simulink model "closed_loop5"  (R2012b)
settings: Solver=ode3  StartTime=0.0  StopTime=t_total+100  FixedStep=0.001  RelTol=1e-3
values from neighbouring files (symbols this model uses):
  a = D/(8*(t1^2)*(n^2))    [Craneparameters.m]    (also in Craneparameters2.m = 0.428041999052; Craneparameters3.m = 0.428041999052; Craneparameters4.m = 0.5; Craneparameters5.m = 0.428041999052)
  a2 = D/(2*(4*p+1)*p*(t1^2))    [Craneparameters2.m]    (also in Craneparameters3.m = D/(2*(4*n+5)*(n+1)*(t1^2)); Craneparameters5.m = D/(2*(4*n+5)*(n+1)*(t1^2)))
  g = 9.81    [Craneparameters.m]    (also in Craneparameters2.m; Craneparameters3.m; Craneparameters4.m; Craneparameters5.m)
  K = 2/w    [Craneparameters4.m]    (also in Craneparameters5.m; Prototype_parameters.m; Slidingmode.m)
  l = 40    [Craneparameters.m]    (also in Craneparameters2.m; Craneparameters3.m; Craneparameters4.m; Craneparameters5.m)
  M = 26*10^3    (= 26000)    [Craneparameters.m]    (also in Craneparameters2.m; Craneparameters3.m; Craneparameters4.m; Craneparameters5.m)
  m = 67.3*10^3    (= 67300)    [Craneparameters.m]    (also in Craneparameters2.m; Craneparameters3.m; Craneparameters4.m; Craneparameters5.m)
  T = 2*pi/w    [Craneparameters.m]    (also in Craneparameters2.m; Craneparameters3.m; Craneparameters4.m; Craneparameters5.m)
  T1 = n*T    [Craneparameters.m]    (also in Craneparameters2.m; Craneparameters3.m; Craneparameters4.m = t1; Craneparameters5.m)
  T2 = n*T+t2    [Craneparameters.m]    (also in Craneparameters2.m; Craneparameters3.m = (n+1)*T; Craneparameters4.m = t1+t2; Craneparameters5.m = (n+1)*T)
  T3 = (n+1)*T+t2    [Craneparameters3.m]    (also in Craneparameters5.m)
  T4 = (n+2)*T+t2    [Craneparameters3.m]    (also in Craneparameters5.m)
  t_total = 2*n*T + t2    [Craneparameters.m]    (also in Craneparameters2.m = t_total2; Craneparameters3.m = 2*(n+1)*T + t2; Craneparameters4.m = T2+t1; Craneparameters5.m = 2*(n+1)*T + t2)
libraries: simulink x2
settings Model: Creator=mchusr  LastModifiedBy=mchusr

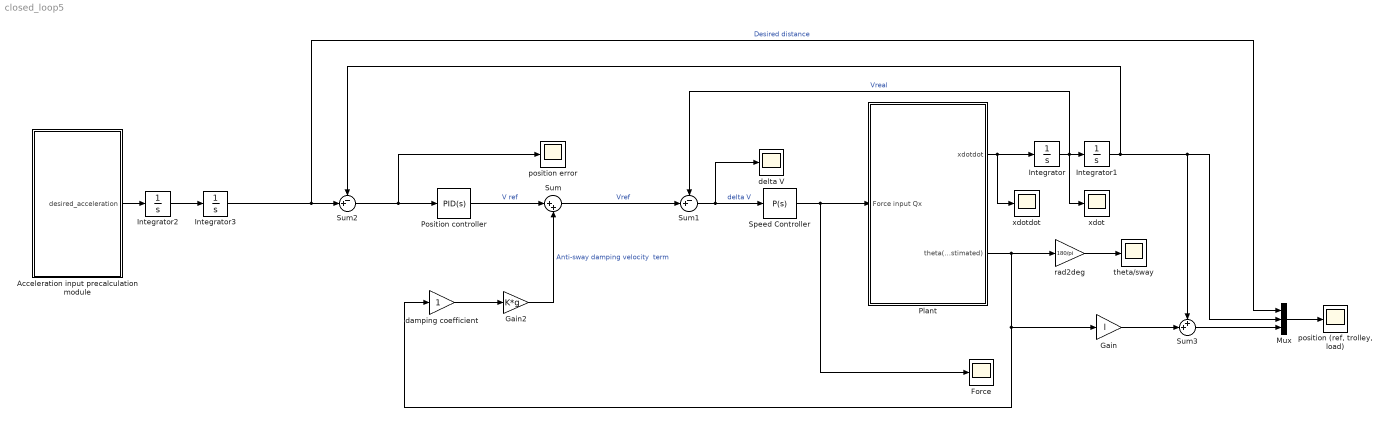
== system closed_loop5 ==
  Acceleration input precalculation module : Subsystem
  Force : Scope
      settings: TimeRange=105  YMin=-600000  YMax=100000  SaveName=xdotdot1
  Gain : Gain  Gain=l
  Gain2 : Gain  Gain=K*g
  Integrator{,1..3} (4 alike) : Integrator
  Mux : Mux  Inputs=3
  Plant : Subsystem
  Position controller : simulink/Continuous/PID Controller  Controller=PID  TimeDomain=Continuous-time  SampleTime=1  IntegratorMethod=Forward Euler  FilterMethod=Forward Euler  Form=Parallel  P=3  I=0.08  D=0.4  N=100  InitialConditionSource=internal  InitialConditionForIntegrator=0  InitialConditionForFilter=0  ExternalReset=none  LimitOutput=off  UpperSaturationLimit=inf  LowerSaturationLimit=-inf  LinearizeAsGain=on  AntiWindupMode=none  Kb=1  TrackingMode=off  Kt=1  PParamMin=[]  PParamMax=[]  IParamMin=[]  IParamMax=[]  DParamMin=[]  DParamMax=[]  NParamMin=[]  NParamMax=[]  KbParamMin=[]  KbParamMax=[]  KtParamMin=[]  KtParamMax=[]  POutMin=[]  POutMax=[]  IOutMin=[]  IOutMax=[]  DOutMin=[]  DOutMax=[]  NOutMin=[]  NOutMax=[]  KbOutMin=[]  KbOutMax=[]  KtOutMin=[]  KtOutMax=[]  IntegratorOutMin=[]  IntegratorOutMax=[]  FilterOutMin=[]  FilterOutMax=[]  SumOutMin=[]  SumOutMax=[]  SumI1OutMin=[]  SumI1OutMax=[]  SumI2OutMin=[]  SumI2OutMax=[]  SumI3OutMin=[]  SumI3OutMax=[]  SumDOutMin=[]  SumDOutMax=[]  SaturationOutMin=[]  SaturationOutMax=[]  IntegratorContinuousStateAttributes=''  IntegratorStateMustResolveToSignalObject=off  IntegratorRTWStateStorageClass=Auto  FilterContinuousStateAttributes=''  FilterStateMustResolveToSignalObject=off  FilterRTWStateStorageClass=Auto
  Speed Controller : simulink/Continuous/PID Controller  Controller=P  TimeDomain=Continuous-time  SampleTime=1  IntegratorMethod=Forward Euler  FilterMethod=Forward Euler  Form=Parallel  P=(M+m)  I=10*(M+m)  D=(M+m)  N=100  InitialConditionSource=internal  InitialConditionForIntegrator=0  InitialConditionForFilter=0  ExternalReset=none  LimitOutput=off  UpperSaturationLimit=inf  LowerSaturationLimit=-inf  LinearizeAsGain=on  AntiWindupMode=none  Kb=1  TrackingMode=off  Kt=1  PParamMin=[]  PParamMax=[]  IParamMin=[]  IParamMax=[]  DParamMin=[]  DParamMax=[]  NParamMin=[]  NParamMax=[]  KbParamMin=[]  KbParamMax=[]  KtParamMin=[]  KtParamMax=[]  POutMin=[]  POutMax=[]  IOutMin=[]  IOutMax=[]  DOutMin=[]  DOutMax=[]  NOutMin=[]  NOutMax=[]  KbOutMin=[]  KbOutMax=[]  KtOutMin=[]  KtOutMax=[]  IntegratorOutMin=[]  IntegratorOutMax=[]  FilterOutMin=[]  FilterOutMax=[]  SumOutMin=[]  SumOutMax=[]  SumI1OutMin=[]  SumI1OutMax=[]  SumI2OutMin=[]  SumI2OutMax=[]  SumI3OutMin=[]  SumI3OutMax=[]  SumDOutMin=[]  SumDOutMax=[]  SaturationOutMin=[]  SaturationOutMax=[]  IntegratorContinuousStateAttributes=''  IntegratorStateMustResolveToSignalObject=off  IntegratorRTWStateStorageClass=Auto  FilterContinuousStateAttributes=''  FilterStateMustResolveToSignalObject=off  FilterRTWStateStorageClass=Auto
  Sum : Sum  Inputs=|++
  Sum1 : Sum  Inputs=-+|
  Sum2 : Sum  Inputs=-+|
  Sum3 : Sum  Inputs=++|
  damping coefficient : Gain
  delta V : Scope
      settings: TimeRange=105  YMin=-7.5e-08  YMax=7.5e-08  SaveName=xdotdot3
  "position (ref, trolley, load)" : Scope
      settings: TimeRange=139.097  YMin=98.25  YMax=101.75  SaveName=position2
  position error : Scope
      settings: TimeRange=105  YMin=-0.105  YMax=-0.025  SaveName=xdotdot2
  rad2deg : Gain  Gain=180/pi
  theta/sway : Scope
      settings: YMin=-0.175  YMax=0.175  SaveName=sway2
  xdot : Scope
      settings: TimeRange=64.833  YMin=5.55112e-17  YMax=1.9  SaveName=velocity
  xdotdot : Scope
      settings: TimeRange=105  YMin=-7.5e-08  YMax=7.5e-08  SaveName=xdotdot
  wires:
  Plant/1(xdotdot) -> Integrator/1, xdotdot/1
  Integrator/1 -> Sum1/1, xdot/1, Integrator1/1  "Vreal"
  Integrator1/1 -> Mux/2, Sum3/1, Sum2/1
  Plant/2(theta(estimated)) -> rad2deg/1, damping coefficient/1, Gain/1
  Speed Controller/1 -> Plant/1(Force input Qx), Force/1
  Position controller/1 -> Sum/1  "V ref"
  Gain2/1 -> Sum/2  "Anti-sway damping velocity  term"
  damping coefficient/1 -> Gain2/1
  Sum/1 -> Sum1/2  "Vref"
  Sum1/1 -> delta V/1, Speed Controller/1  "delta V"
  Sum2/1 -> position error/1, Position controller/1
  Integrator3/1 -> Sum2/2, Mux/1  "Desired distance"
  rad2deg/1 -> theta/sway/1
  Gain/1 -> Sum3/2
  Sum3/1 -> Mux/3
  Mux/1 -> "position (ref, trolley, load)"/1
  Acceleration input precalculation module/1(desired_acceleration) -> Integrator2/1
  Integrator2/1 -> Integrator3/1

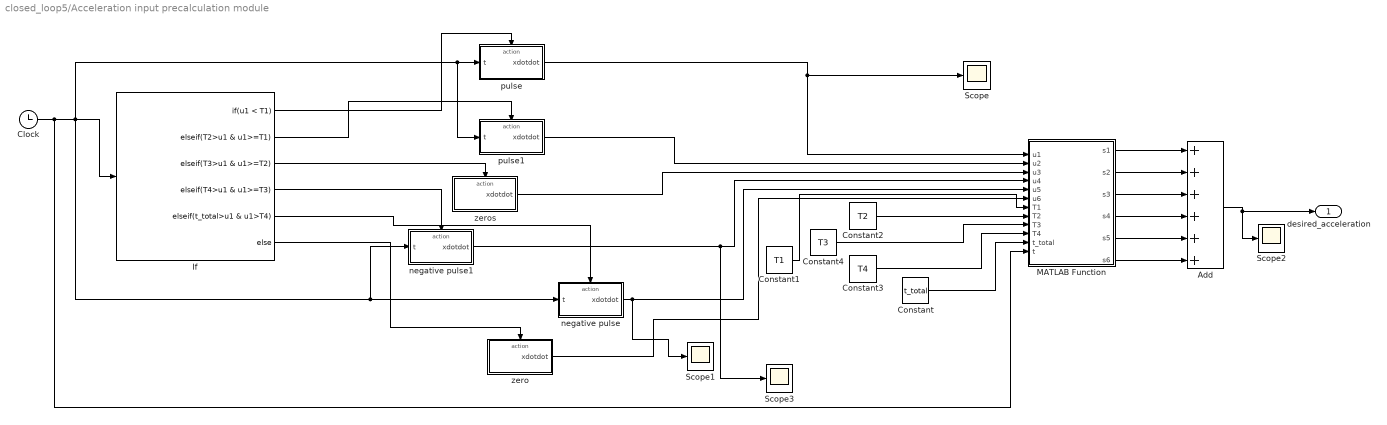
== system closed_loop5/Acceleration input precalculation module ==
  Add : Sum  Inputs=++++++
  Clock : Clock
  Constant : Constant  Value=t_total
  Constant1 : Constant  Value=T1
  Constant2 : Constant  Value=T2
  Constant3 : Constant  Value=T4
  Constant4 : Constant  Value=T3
  If : If  IfExpression=u1 < T1  ElseIfExpressions=T2>u1 & u1>=T1, T3>u1 & u1>=T2, T4>u1 & u1>=T3, t_total>u1 & u1>T4  ZeroCross=off
  MATLAB Function : MATLAB Function  TreatAsAtomicUnit=on
  Scope{,1..3} (4 alike) : Scope
      Scope settings: SaveName=ScopeData4
      Scope1 settings: SaveName=ScopeData5
      Scope2 settings: SaveName=ScopeData6
  negative pulse : Subsystem  TreatAsAtomicUnit=on
  negative pulse1 : Subsystem  TreatAsAtomicUnit=on
  pulse : Subsystem  TreatAsAtomicUnit=on
  pulse1 : Subsystem  TreatAsAtomicUnit=on
  "zero " : Subsystem  TreatAsAtomicUnit=on
  zeros : Subsystem  TreatAsAtomicUnit=on
  desired_acceleration : Outport
  wires:
  If/1 -> pulse/Action
  Clock/1 -> MATLAB Function/12(t), pulse1/1(t), pulse/1(t), negative pulse1/1(t), negative pulse/1(t), If/1
  Add/1 -> Scope2/1, desired_acceleration/1
  pulse/1(xdotdot) -> MATLAB Function/1(u1), Scope/1
  MATLAB Function/1(s1) -> Add/1
  MATLAB Function/2(s2) -> Add/2
  MATLAB Function/3(s3) -> Add/3
  MATLAB Function/4(s4) -> Add/4
  Constant1/1 -> MATLAB Function/7(T1)
  Constant/1 -> MATLAB Function/11(t_total)
  MATLAB Function/5(s5) -> Add/5
  Constant2/1 -> MATLAB Function/8(T2)
  Constant4/1 -> MATLAB Function/9(T3)
  Constant3/1 -> MATLAB Function/10(T4)
  If/2 -> pulse1/Action
  pulse1/1(xdotdot) -> MATLAB Function/2(u2)
  If/3 -> zeros/Action
  zeros/1(xdotdot) -> MATLAB Function/3(u3)
  If/4 -> negative pulse1/Action
  If/5 -> negative pulse/Action
  negative pulse1/1(xdotdot) -> Scope3/1, MATLAB Function/4(u4)
  negative pulse/1(xdotdot) -> Scope1/1, MATLAB Function/5(u5)
  If/6 -> "zero "/Action
  "zero "/1(xdotdot) -> MATLAB Function/6(u6)
  MATLAB Function/6(s6) -> Add/6

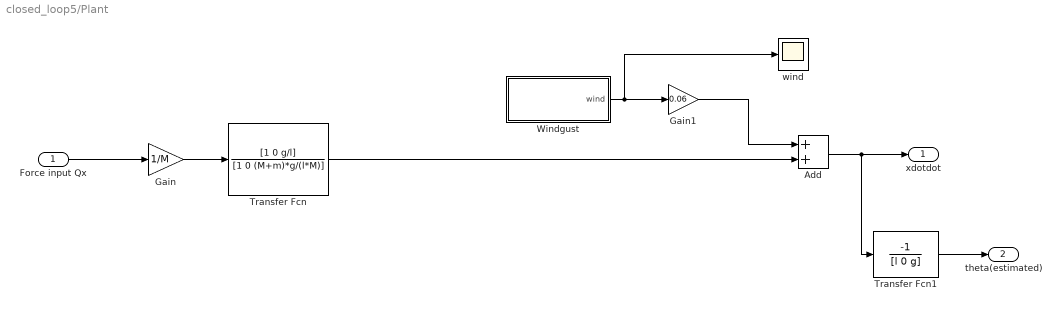
== system closed_loop5/Plant ==
  Force input Qx : Inport
  Add : Sum
  Gain : Gain  Gain=1/M
  Gain1 : Gain  Gain=0.06
  Transfer Fcn : TransferFcn  Numerator=[1 0 g/l]  Denominator=[1 0 (M+m)*g/(l*M)]
  Transfer Fcn1 : TransferFcn  Numerator=[-1]  Denominator=[l 0 g]
  Windgust : Subsystem
  wind : Scope
      settings: SaveName=wind
  xdotdot : Outport
  theta(estimated) : Outport  Port=2
  wires:
  Force input Qx/1 -> Gain/1
  Gain/1 -> Transfer Fcn/1
  Transfer Fcn/1 -> Add/2
  Transfer Fcn1/1 -> theta(estimated)/1
  Windgust/1(wind) -> wind/1, Gain1/1
  Add/1 -> Transfer Fcn1/1, xdotdot/1
  Gain1/1 -> Add/1

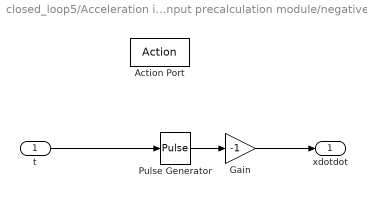
== system closed_loop5/Acceleration input precalculation module/negative pulse ==
  t : Inport
  Action Port : ActionPort  ActionType=elseif
  Gain : Gain  Gain=-1
  Pulse Generator : DiscretePulseGenerator  PulseType=Time based  TimeSource=Use external signal  Amplitude=a  Period=T/2  PulseWidth=50  PhaseDelay=T4  SampleTime=0.001
  xdotdot : Outport
  wires:
  t/1 -> Pulse Generator/1
  Pulse Generator/1 -> Gain/1
  Gain/1 -> xdotdot/1

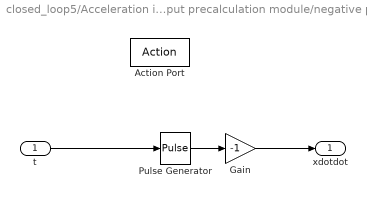
== system closed_loop5/Acceleration input precalculation module/negative pulse1 ==
  t : Inport
  Action Port : ActionPort  ActionType=elseif
  Gain : Gain  Gain=-1
  Pulse Generator : DiscretePulseGenerator  PulseType=Time based  TimeSource=Use external signal  Amplitude=a2  Period=T/2  PulseWidth=50  PhaseDelay=T3  SampleTime=0.001
  xdotdot : Outport
  wires:
  t/1 -> Pulse Generator/1
  Pulse Generator/1 -> Gain/1
  Gain/1 -> xdotdot/1

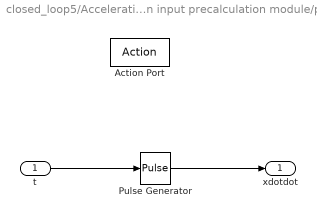
== system closed_loop5/Acceleration input precalculation module/pulse ==
  t : Inport
  Action Port : ActionPort  ActionType=then
  Pulse Generator : DiscretePulseGenerator  PulseType=Time based  TimeSource=Use external signal  Amplitude=a  Period=T/2  PulseWidth=50  SampleTime=0.001
  xdotdot : Outport
  wires:
  Pulse Generator/1 -> xdotdot/1
  t/1 -> Pulse Generator/1

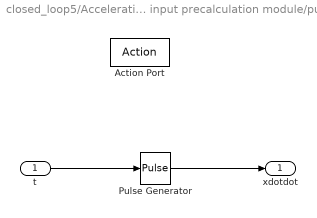
== system closed_loop5/Acceleration input precalculation module/pulse1 ==
  t : Inport
  Action Port : ActionPort  ActionType=elseif
  Pulse Generator : DiscretePulseGenerator  PulseType=Time based  TimeSource=Use external signal  Amplitude=a2  Period=T/2  PulseWidth=50  PhaseDelay=T1  SampleTime=0.001
  xdotdot : Outport
  wires:
  Pulse Generator/1 -> xdotdot/1
  t/1 -> Pulse Generator/1

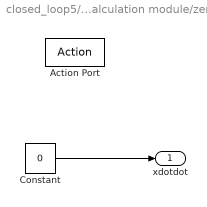
== system closed_loop5/Acceleration input precalculation module/zero  ==
  Action Port : ActionPort  ActionType=else
  Constant : Constant  Value=0
  xdotdot : Outport
  wires:
  Constant/1 -> xdotdot/1

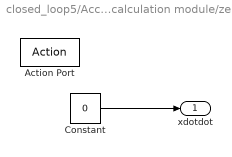
== system closed_loop5/Acceleration input precalculation module/zeros ==
  Action Port : ActionPort  ActionType=elseif
  Constant : Constant  Value=0
  xdotdot : Outport
  wires:
  Constant/1 -> xdotdot/1

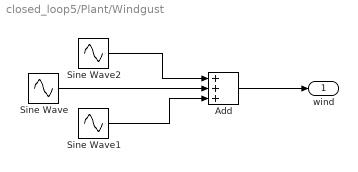
== system closed_loop5/Plant/Windgust ==
  Add : Sum  Inputs=+++
  Sine Wave : Sin  Amplitude=5  Frequency=0.2  SampleTime=0
  Sine Wave1 : Sin  Amplitude=3  Frequency=0.3  Phase=1  SampleTime=0
  Sine Wave2 : Sin  Phase=2.04  SampleTime=0
  wind : Outport
  wires:
  Sine Wave2/1 -> Add/1
  Sine Wave/1 -> Add/2
  Sine Wave1/1 -> Add/3
  Add/1 -> wind/1

== matlab function closed_loop5/Acceleration input precalculation module/MATLAB Function ==
  data: u1 input; s1 output; u2 input; u3 input; u4 input; u5 input; u6 input; T1 input; T2 input; T3 input; T4 input; t_total input; s2 output; s3 output; s4 output; t input; s5 output; s6 output
function [s1, s2, s3, s4, s5, s6] = filter(u1, u2, u3, u4, u5, u6, T1, T2, T3, T4, t_total, t)

if t<T1
    s1 = u1;
else
    s1=0;
end

if t<T2
    s2 = u2;
else
    s2=0;
end

s3=u3;

if t<T4
    s4 = u4;
else
    s4=0;
end

if t<t_total
    s5 = u5;
else
    s5=0;
end



s6=u6;




end
